simulink model "CotroladoresSeguidor"  (R2025a)
settings: Solver=VariableStepAuto  StartTime=0.0  StopTime=1  RelTol=1e-3
values from neighbouring files (symbols this model uses):
  denominador = den_d    [Control Planta.m]    (also in Control_Planta.m)
  numerador = num_d    [Control Planta.m]    (also in Control_Planta.m)
  r0 = 62.5219    [Control Planta.m]    (also in Control_Planta.m)
  r1 = -148.912    [Control Planta.m]    (also in Control_Planta.m)
  r2 = 147.642    [Control Planta.m]    (also in Control_Planta.m)
  s0 = 0.139719    [Control Planta.m]    (also in Control_Planta.m)
undefined symbols (not defined in the file or in its folder): dspblkCoreblockFVToolHelper, gcbh

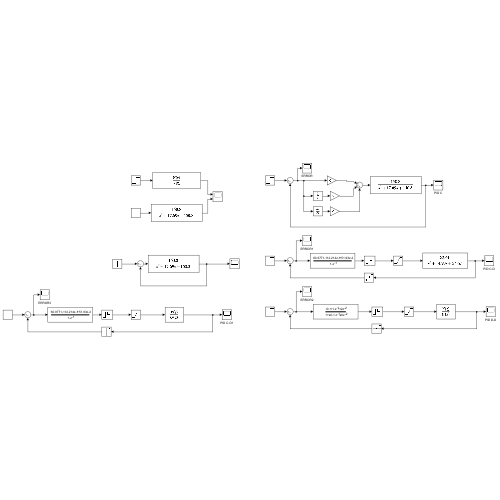
[thumbnail: Simulink's stored preview of the top-level diagram]
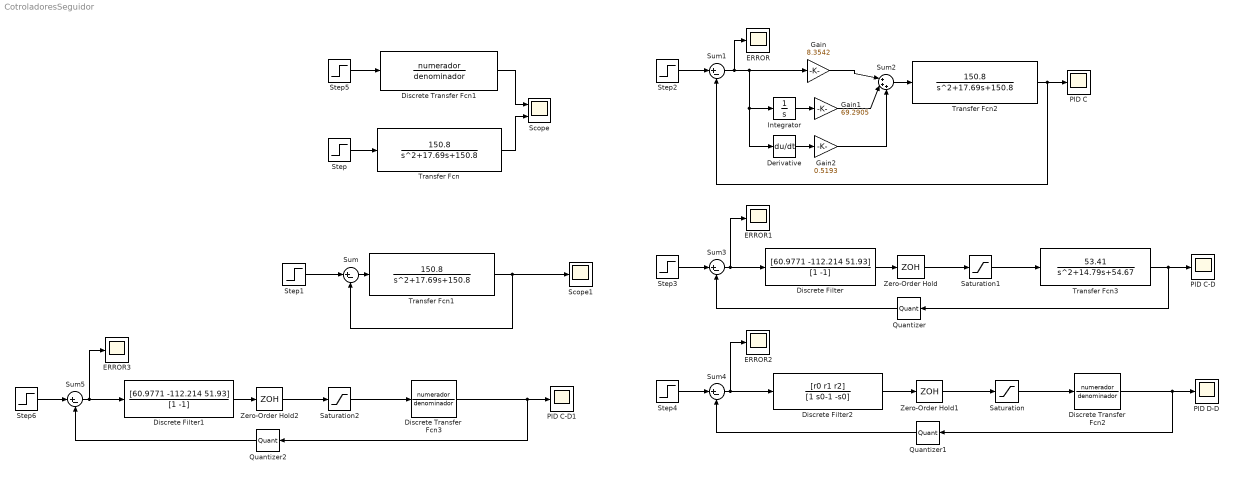
== system CotroladoresSeguidor ==
  Derivative : Derivative
  Discrete Transfer Fcn1 : DiscreteTransferFcn  LoadFcn=dspblkCoreblockFVToolHelper(gcbh,'load');  Numerator=numerador  Denominator=denominador
  Discrete Transfer Fcn2 : DiscreteTransferFcn  LoadFcn=dspblkCoreblockFVToolHelper(gcbh,'load');  Numerator=numerador  Denominator=denominador
  Discrete Transfer Fcn3 : DiscreteTransferFcn  LoadFcn=dspblkCoreblockFVToolHelper(gcbh,'load');  Numerator=numerador  Denominator=denominador
  Discrete Filter : DiscreteFilter  LoadFcn=dspblkCoreblockFVToolHelper(gcbh,'load');  Numerator=[60.9771 -112.214 51.93]  Denominator=[1 -1]
  Discrete Filter1 : DiscreteFilter  LoadFcn=dspblkCoreblockFVToolHelper(gcbh,'load');  Numerator=[60.9771 -112.214 51.93]  Denominator=[1 -1]
  Discrete Filter2 : DiscreteFilter  LoadFcn=dspblkCoreblockFVToolHelper(gcbh,'load');  Numerator=[r0 r1 r2]  Denominator=[1 s0-1 -s0]
  ERROR{,1..3} (4 alike) : Scope
  Gain : Gain  Gain=8.3542
  Gain1 : Gain  Gain=69.2905
  Gain2 : Gain  Gain=0.5193
  Integrator : Integrator
  PID C : Scope
  PID C-D : Scope
  PID C-D1 : Scope
  PID D-D : Scope
  Quantizer : Quantizer  QuantizationInterval=3.3/4095
  Quantizer1 : Quantizer  QuantizationInterval=3.3/4095
  Quantizer2 : Quantizer  QuantizationInterval=3.3/4095
  Saturation : Saturate  UpperLimit=14  LowerLimit=-14
  Saturation1 : Saturate  UpperLimit=14  LowerLimit=-14
  Saturation2 : Saturate  UpperLimit=14  LowerLimit=-14
  Scope : Scope  NumInputPorts=2
  Scope1 : Scope
  Step{,1..6} (7 alike) : Step  Time=0  SampleTime=0
  Sum{,1,3..5} (5 alike) : Sum  Inputs=|+-
  Sum2 : Sum  Inputs=|+++
  Transfer Fcn : TransferFcn  Numerator=[150.8]  Denominator=[1 17.69 150.8]
  Transfer Fcn1 : TransferFcn  Numerator=[150.8]  Denominator=[1 17.69 150.8]
  Transfer Fcn2 : TransferFcn  Numerator=[150.8]  Denominator=[1 17.69 150.8]
  Transfer Fcn3 : TransferFcn  Numerator=[53.41]  Denominator=[1 14.79 54.67]
  Zero-Order Hold : ZeroOrderHold  SampleTime=0.01
  Zero-Order Hold1 : ZeroOrderHold  SampleTime=0.01
  Zero-Order Hold2 : ZeroOrderHold  SampleTime=0.01
  wires:
  Step/1 -> Transfer Fcn/1
  Sum/1 -> Transfer Fcn1/1
  Step1/1 -> Sum/1
  Transfer Fcn1/1 -> Scope1/1, Sum/2
  Integrator/1 -> Gain1/1
  Derivative/1 -> Gain2/1
  Gain/1 -> Sum2/1
  Gain1/1 -> Sum2/2
  Gain2/1 -> Sum2/3
  Step2/1 -> Sum1/1
  Sum2/1 -> Transfer Fcn2/1
  Transfer Fcn2/1 -> PID C/1, Sum1/2
  Sum1/1 -> ERROR/1, Derivative/1, Integrator/1, Gain/1
  Step3/1 -> Sum3/1
  Sum3/1 -> ERROR1/1, Discrete Filter/1
  Discrete Filter/1 -> Zero-Order Hold/1
  Zero-Order Hold/1 -> Saturation1/1
  Quantizer/1 -> Sum3/2
  Transfer Fcn3/1 -> PID C-D/1, Quantizer/1
  Zero-Order Hold1/1 -> Saturation/1
  Discrete Transfer Fcn2/1 -> PID D-D/1, Quantizer1/1
  Sum4/1 -> Discrete Filter2/1, ERROR2/1
  Step4/1 -> Sum4/1
  Quantizer1/1 -> Sum4/2
  Discrete Filter2/1 -> Zero-Order Hold1/1
  Transfer Fcn/1 -> Scope/2
  Saturation/1 -> Discrete Transfer Fcn2/1
  Saturation1/1 -> Transfer Fcn3/1
  Step5/1 -> Discrete Transfer Fcn1/1
  Discrete Transfer Fcn1/1 -> Scope/1
  Saturation2/1 -> Discrete Transfer Fcn3/1
  Discrete Transfer Fcn3/1 -> Quantizer2/1, PID C-D1/1
  Quantizer2/1 -> Sum5/2
  Zero-Order Hold2/1 -> Saturation2/1
  Discrete Filter1/1 -> Zero-Order Hold2/1
  Sum5/1 -> Discrete Filter1/1, ERROR3/1
  Step6/1 -> Sum5/1
